simulink model "q2_state1_pid"  (R2021b)
settings: Solver=VariableStepAuto  StartTime=0.0  StopTime=400  RelTol=1e-3
undefined symbols (not defined in the file or in its folder): Kd, Ki, Kp
settings Model: Creator=Reyhaneh  LastModifiedBy=Reyhaneh

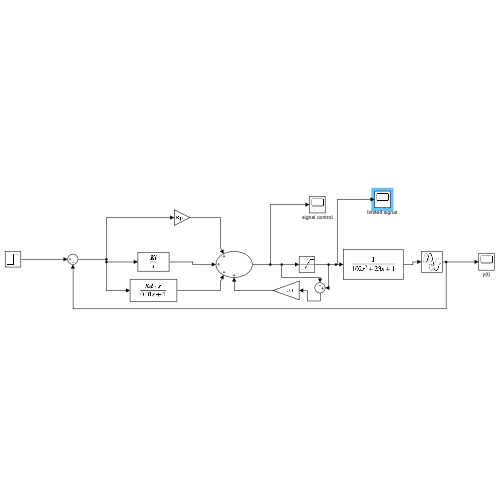
[thumbnail: Simulink's stored preview of the top-level diagram]
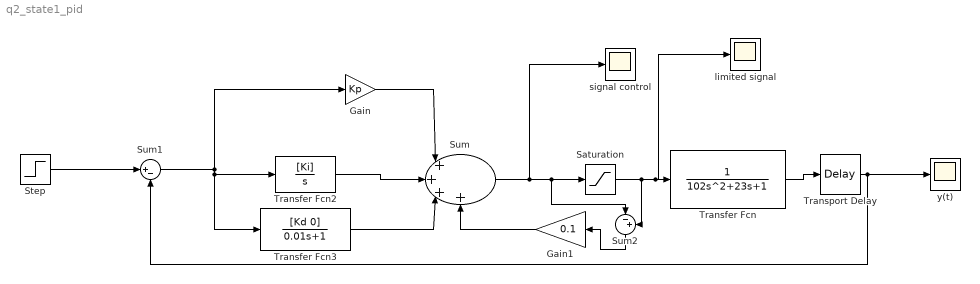
== system q2_state1_pid ==
  Gain : Gain  Gain=Kp
  Gain1 : Gain  Gain=0.1
  Saturation : Saturate  UpperLimit=15  LowerLimit=-15
  Step : Step  Time=0  SampleTime=0
  Sum : Sum  Inputs=|++++
  Sum1 : Sum  Inputs=|+-
  Sum2 : Sum  Inputs=|-+
  Transfer Fcn : TransferFcn  Denominator=[102 23 1]
  Transfer Fcn2 : TransferFcn  Numerator=[Ki]  Denominator=[1 0]
  Transfer Fcn3 : TransferFcn  Numerator=[Kd 0]  Denominator=[0.01 1]
  Transport Delay : TransportDelay  DelayTime=30
  limited signal : Scope
  signal control : Scope
  y(t) : Scope
  wires:
  Transport Delay/1 -> Sum1/2, y(t)/1
  Transfer Fcn2/1 -> Sum/2
  Gain/1 -> Sum/1
  Sum/1 -> signal control/1, Sum2/1, Saturation/1
  Step/1 -> Sum1/1
  Transfer Fcn/1 -> Transport Delay/1
  Sum1/1 -> Transfer Fcn3/1, Transfer Fcn2/1, Gain/1
  Transfer Fcn3/1 -> Sum/3
  Saturation/1 -> limited signal/1, Transfer Fcn/1, Sum2/2
  Sum2/1 -> Gain1/1
  Gain1/1 -> Sum/4
